simulink model "ECE411_Project_WindTorquebaik"  (R2022a)
settings: Solver=VariableStepAuto  StartTime=0.0  StopTime=1.5  RelTol=1e-3
libraries: simulink x1
settings Model: Creator=DiggerPC  LastModifiedBy=MRGOAT
settings DebuggingCC: UnconnectedInputMsg=warning  UnconnectedOutputMsg=warning  UnconnectedLineMsg=warning
settings RTWCC: DLArmComputeVersion=19.05

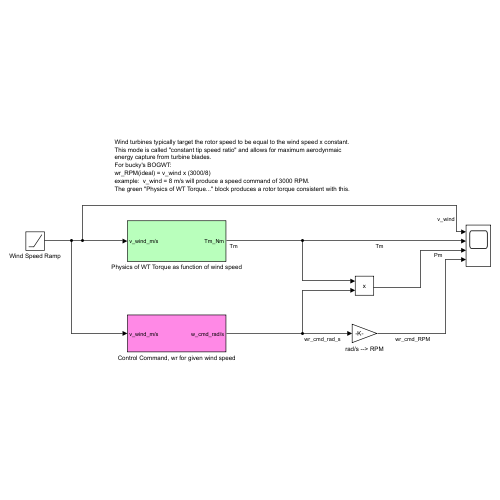
[thumbnail: Simulink's stored preview of the top-level diagram]
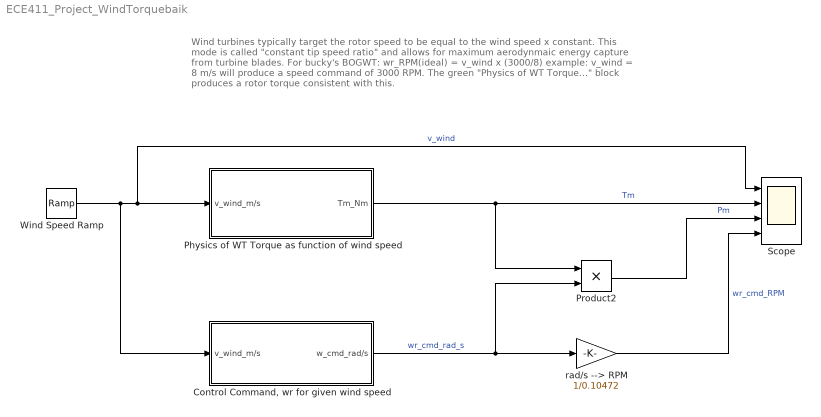
== system ECE411_Project_WindTorquebaik ==
  note: Wind turbines typically target the rotor speed to be equal to the wind speed x constant.  This mode is called "constant tip speed ratio" and allows for maximum aerodynmaic energy capture from turbine blades.
      | For bucky's BOGWT:
      | wr_RPM(ideal) = v_wind x (3000/8)
      | example:  v_wind = 8 m/s will produce a speed command of 3000 RPM.
      | The green "Physics of WT Torque..." block produces a rotor torque consistent with this.
  "Control Command, wr for given wind speed" : Subsystem
  Physics of WT Torque as function of wind speed : Subsystem
  Product2 : Product
  Scope : Scope  NumInputPorts=4
  Wind Speed Ramp : simulink/Sources/Ramp  slope=8  start=0  InitialOutput=0
  rad/s --> RPM : Gain  Gain=1/0.10472
  wires:
  Wind Speed Ramp/1 -> Scope/1, Physics of WT Torque as function of wind speed/1(v_wind_m/s), "Control Command, wr for given wind speed"/1(v_wind_m/s)  "v_wind"
  Product2/1 -> Scope/3  "Pm"
  "Control Command, wr for given wind speed"/1(w_cmd_rad/s) -> rad/s --> RPM/1, Product2/2  "wr_cmd_rad_s"
  Physics of WT Torque as function of wind speed/1(Tm_Nm) -> Scope/2, Product2/1  "Tm"
  rad/s --> RPM/1 -> Scope/4  "wr_cmd_RPM"

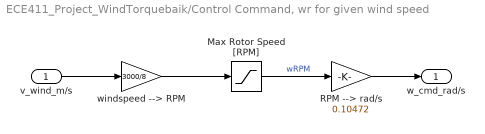
== system ECE411_Project_WindTorquebaik/Control Command, wr for given wind speed ==
  v_wind_m/s : Inport
  Max Rotor Speed [RPM] : Saturate  UpperLimit=3750  LowerLimit=0
  RPM --> rad/s : Gain  Gain=0.10472
  windspeed --> RPM : Gain  Gain=3000/8
  w_cmd_rad/s : Outport
  wires:
  v_wind_m/s/1 -> windspeed --> RPM/1
  Max Rotor Speed [RPM]/1 -> RPM --> rad/s/1  "wRPM"
  windspeed --> RPM/1 -> Max Rotor Speed [RPM]/1
  RPM --> rad/s/1 -> w_cmd_rad/s/1

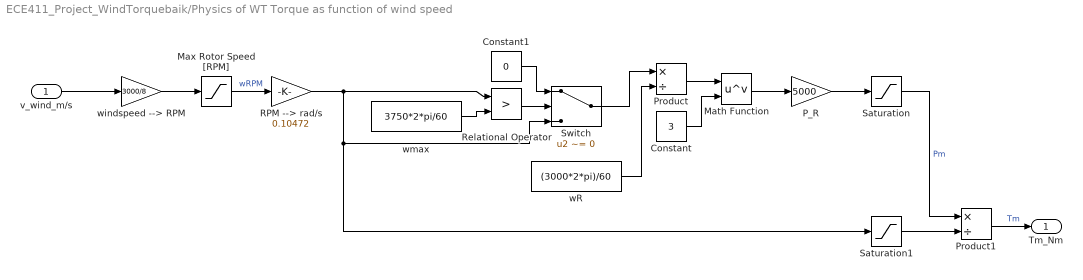
== system ECE411_Project_WindTorquebaik/Physics of WT Torque as function of wind speed ==
  v_wind_m/s : Inport
  Constant : Constant  Value=3
  Constant1 : Constant  Value=0
  Math Function : Math  Operator=pow
  Max Rotor Speed [RPM] : Saturate  UpperLimit=3750  LowerLimit=0
  P_R : Gain  Gain=5000
  Product : Product  Inputs=*/
  Product1 : Product  Inputs=*/
  RPM --> rad/s : Gain  Gain=0.10472
  Relational Operator : RelationalOperator  Operator=>  OutDataTypeStr=boolean  RndMeth=Simplest  InputSameDT=off
  Saturation : Saturate  UpperLimit=5000  LowerLimit=0
  Saturation1 : Saturate  UpperLimit=3750*2*pi/60  LowerLimit=1e-6
  Switch : Switch  Criteria=u2 ~= 0  SaturateOnIntegerOverflow=off  InputSameDT=off
  wR : Constant  Value=(3000*2*pi)/60
  windspeed --> RPM : Gain  Gain=3000/8
  wmax : Constant  Value=3750*2*pi/60
  Tm_Nm : Outport
  wires:
  Saturation/1 -> Product1/1  "Pm"
  Math Function/1 -> P_R/1
  Max Rotor Speed [RPM]/1 -> RPM --> rad/s/1  "wRPM"
  Relational Operator/1 -> Switch/2
  Product/1 -> Math Function/1
  windspeed --> RPM/1 -> Max Rotor Speed [RPM]/1
  Product1/1 -> Tm_Nm/1  "Tm"
  Switch/1 -> Product/1
  P_R/1 -> Saturation/1
  v_wind_m/s/1 -> windspeed --> RPM/1
  RPM --> rad/s/1 -> Saturation1/1, Switch/3, Relational Operator/1
  wmax/1 -> Relational Operator/2
  Constant1/1 -> Switch/1
  Constant/1 -> Math Function/2
  Saturation1/1 -> Product1/2
  wR/1 -> Product/2
